simulink model "icl_control"  (R2021a)
settings: Solver=FixedStepAuto  StartTime=0.0  StopTime=inf  FixedStep=Ts  RelTol=1e-3  EnableMultiTasking=on
InitFcn:
  | Ts = 0.001; % sample time
  | Tc = 0.008; % controller sample time
settings Model: SimulationMode=external  ExtModeEnableFloating=off  ExplicitPartitioning=on  Creator=zhaoyx  LastModifiedBy=icl-baby
settings SolverCC: ConcurrentTasks=on  AlgebraicLoopSolver=TrustRegion  PositivePriorityOrder=on  AutoInsertRateTranBlk=on  InsertRTBMode=Never (minimum delay)
settings DataIOCC: SaveFormat=StructureWithTime  ReturnWorkspaceOutputs=off
settings OptimizationCC: BlockReduction=off  DefaultParameterBehavior=Inlined  OptimizeBlockIOStorage=off  BufferReuse=off  GlobalBufferReuse=off  ExpressionFolding=off  LocalBlockOutputs=off  OptimizeDataStoreBuffers=off  BusAssignmentInplaceUpdate=off
settings DebuggingCC: TasksWithSamePriorityMsg=none  SFMachineParentedDataDiag=warning  ArithmeticOperatorsInVariantConditions=warning
settings HardwareCC: ProdBitPerLong=64  ProdLongLongMode=on  ProdHWDeviceType=Intel->x86-64 (Linux 64)
settings SFSimCC: CustomCodeUndefinedFunction=UseInterfaceOnly
settings RTWCC: Description=Simulink Real-Time  SystemTargetFile=slrealtime.tlc  TemplateMakefile=slrealtime_default_tmf  Toolchain=Simulink Real-Time Toolchain  BuildConfiguration=Faster Runs  CodeExecutionProfiling=on  TargetLang=C++
settings CodeAppCC: MaxIdLength=95

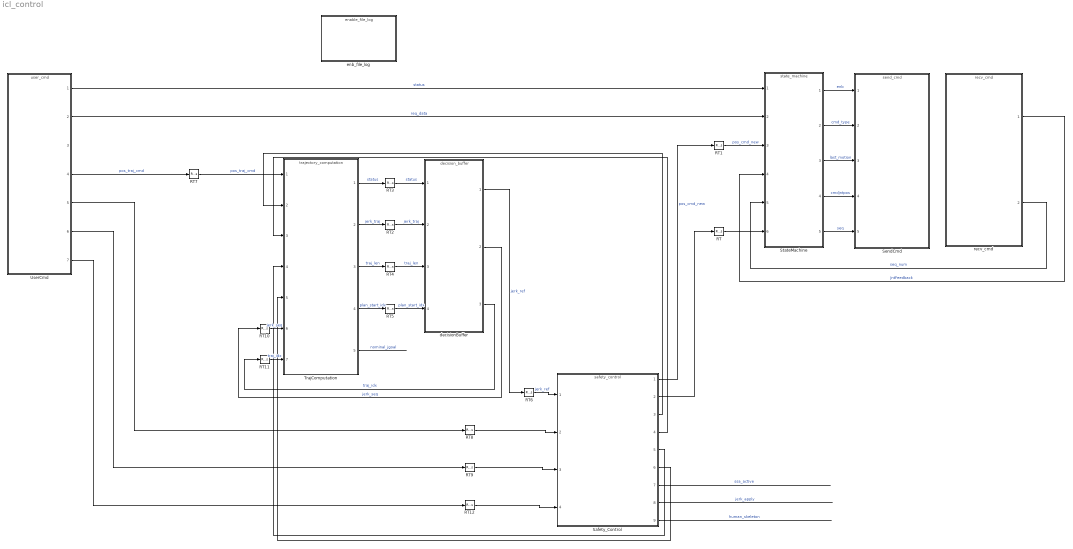
== system icl_control ==
  RT{,1..5} (6 alike) : RateTransition  Deterministic=off  OutPortSampleTime=0.001
  RT{6..12} (7 alike) : RateTransition  Deterministic=off  OutPortSampleTime=0.008
  Safety_Control : ModelReference  ModelNameDialog=safety_control.slx  SimulationMode=Normal  ModelReferenceVersion=1.580
  SendCmd : ModelReference  ModelNameDialog=send_cmd.slx  SimulationMode=Normal  ModelReferenceVersion=1.14
  StateMachine : ModelReference  ModelNameDialog=state_machine.slx  SimulationMode=Normal  ModelReferenceVersion=1.87
  TrajComputation : ModelReference  ModelNameDialog=trajectory_computation.slx  SimulationMode=Normal  ModelReferenceVersion=1.226
  UserCmd : ModelReference  ModelNameDialog=user_cmd.slx  SimulationMode=Normal  ModelReferenceVersion=1.25
  decisionBuffer : ModelReference  ModelNameDialog=decision_buffer.slx  SimulationMode=Normal  ModelReferenceVersion=1.204
  enb_file_log : ModelReference  ModelNameDialog=enable_file_log.slx  SimulationMode=Normal  ModelReferenceVersion=1.2
  recv_cmd : ModelReference  ModelNameDialog=recv_cmd.slx  SimulationMode=Normal  ModelReferenceVersion=1.7
  wires:
  StateMachine/1 -> SendCmd/1  "enb"
  StateMachine/2 -> SendCmd/2  "cmd_type"
  StateMachine/5 -> SendCmd/5  "seq"
  StateMachine/3 -> SendCmd/3  "last_motion"
  StateMachine/4 -> SendCmd/4  "cmdjntpos"
  UserCmd/1 -> StateMachine/1  "status"
  UserCmd/2 -> StateMachine/2  "req_data"
  recv_cmd/1 -> StateMachine/4  "JntFeedback"
  recv_cmd/2 -> StateMachine/5  "seq_num"
  TrajComputation/1 -> RT3/1  "status"
  decisionBuffer/1 -> RT6/1  "jerk_ref"
  TrajComputation/2 -> RT2/1  "jerk_traj"
  TrajComputation/3 -> RT4/1  "traj_len"
  UserCmd/4 -> RT7/1  "pos_traj_cmd"
  TrajComputation/4 -> RT5/1  "plan_start_idx"
  RT2/1 -> decisionBuffer/2  "jerk_traj"
  RT3/1 -> decisionBuffer/1  "status"
  RT4/1 -> decisionBuffer/3  "traj_len"
  RT5/1 -> decisionBuffer/4  "plan_start_idx"
  RT7/1 -> TrajComputation/1  "pos_traj_cmd"
  Safety_Control/5 -> TrajComputation/4
  UserCmd/5 -> RT8/1
  UserCmd/6 -> RT9/1
  decisionBuffer/2 -> RT10/1  "jerk_seq"
  decisionBuffer/3 -> RT11/1  "traj_idx"
  Safety_Control/1 -> RT1/1  "pos_cmd_new"
  Safety_Control/2 -> RT/1
  Safety_Control/3 -> TrajComputation/2
  Safety_Control/4 -> TrajComputation/3
  Safety_Control/6 -> TrajComputation/5
  UserCmd/7 -> RT12/1
  Safety_Control/8 -> ?  "jerk_apply"
  Safety_Control/7 -> ?  "ssa_active"
  RT/1 -> StateMachine/6
  RT1/1 -> StateMachine/3  "pos_cmd_new"
  RT6/1 -> Safety_Control/1  "jerk_ref"
  RT8/1 -> Safety_Control/2
  RT9/1 -> Safety_Control/3
  RT10/1 -> TrajComputation/6  "jerk_seq"
  RT11/1 -> TrajComputation/7  "traj_idx"
  RT12/1 -> Safety_Control/4
  TrajComputation/5 -> ?  "nominal_jgoal"
  Safety_Control/9 -> ?  "human_skeleton"
